simulink model "item2ModeloNLinPS"  (R2017a)
settings: Solver=VariableStepAuto  StartTime=0.0  StopTime=50  RelTol=1e-3
libraries: simulink x4
settings Model: Creator=julia  LastModifiedBy=julia

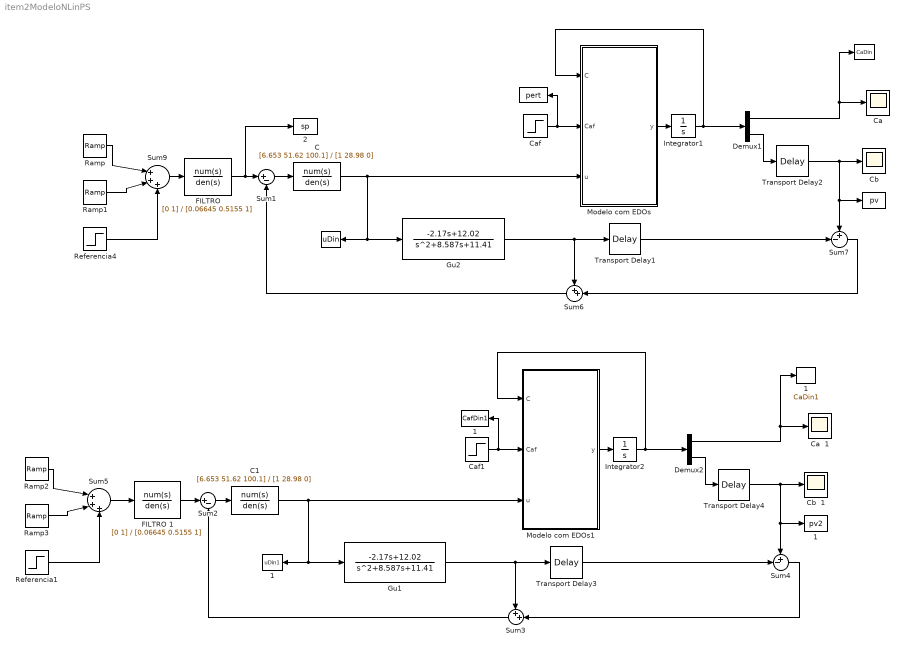
== system item2ModeloNLinPS ==
  "   " : ToWorkspace  VariableName=pv  SaveFormat=Timeseries  SampleTime=-1
  "          " : ToWorkspace  VariableName=pert  SaveFormat=Timeseries  SampleTime=-1
  "                 " : ToWorkspace  VariableName=uDin  SaveFormat=Timeseries  SampleTime=-1
  "                   " : ToWorkspace  VariableName=CaDin  SaveFormat=Timeseries  SampleTime=-1
  "                   1" : ToWorkspace  VariableName=CaDin1  SaveFormat=Timeseries  SampleTime=-1
  "                 1" : ToWorkspace  VariableName=uDin1  SaveFormat=Timeseries  SampleTime=-1
  "          1" : ToWorkspace  VariableName=CafDin1  SaveFormat=Timeseries  SampleTime=-1
  "   1" : ToWorkspace  VariableName=pv2  SaveFormat=Timeseries  SampleTime=-1
  "   2" : ToWorkspace  VariableName=sp  SaveFormat=Timeseries  SampleTime=-1
  C : TransferFcn  Numerator=[6.653 51.62 100.1]  Denominator=[1 28.98 0]
  C1 : TransferFcn  Numerator=[6.653 51.62 100.1]  Denominator=[1 28.98 0]
  "Ca  " : Scope
  Ca  1 : Scope
  Caf : Step  Time=40  Before=5.1  After=5.15  SampleTime=0
  Caf1 : Step  Time=40  Before=5.1  After=5.15  SampleTime=0
  "Cb  " : Scope
  Cb  1 : Scope
  Demux1 : Demux  Outputs=2
  Demux2 : Demux  Outputs=2
  "FILTRO " : TransferFcn  Numerator=[0 1]  Denominator=[0.06645 0.5155 1]
  FILTRO 1 : TransferFcn  Numerator=[0 1]  Denominator=[0.06645 0.5155 1]
  Gu1 : TransferFcn  Numerator=[-2.17 12.02]  Denominator=[1 8.587 11.41]
  Gu2 : TransferFcn  Numerator=[-2.17 12.02]  Denominator=[1 8.587 11.41]
  Integrator1 : Integrator  InitialCondition=[0;0]
  Integrator2 : Integrator  InitialCondition=[0;0]
  Modelo com EDOs : MATLAB Function  TreatAsAtomicUnit=on
  Modelo com EDOs1 : MATLAB Function  TreatAsAtomicUnit=on
  Ramp : simulink/Sources/Ramp  slope=2.345/10  start=0  X0=0
  Ramp1 : simulink/Sources/Ramp  slope=-2.345/10  start=10  X0=0
  Ramp2 : simulink/Sources/Ramp  slope=2.345/10  start=0  X0=0
  Ramp3 : simulink/Sources/Ramp  slope=-2.345/10  start=10  X0=0
  Referencia1 : Step  Time=30  After=0.35  SampleTime=0
  Referencia4 : Step  Time=30  After=0.1  SampleTime=0
  Sum1 : Sum  Inputs=|+-
  Sum2 : Sum  Inputs=|+-
  Sum3 : Sum  Inputs=++|
  Sum4 : Sum  Inputs=+-|
  Sum5 : Sum  Inputs=|+++
  Sum6 : Sum  Inputs=++|
  Sum7 : Sum  Inputs=+-|
  Sum9 : Sum  Inputs=|+++
  Transport Delay{1..4} (4 alike) : TransportDelay  DelayTime=3
  wires:
  Modelo com EDOs/1(y) -> Integrator1/1
  Integrator1/1 -> Modelo com EDOs/1(C), Demux1/1
  Demux1/1 -> "                   "/1, "Ca  "/1
  "FILTRO "/1 -> "   2"/1, Sum1/1
  Sum1/1 -> C/1
  Caf/1 -> "          "/1, Modelo com EDOs/2(Caf)
  Referencia4/1 -> Sum9/3
  Sum9/1 -> "FILTRO "/1
  Ramp1/1 -> Sum9/2
  Ramp/1 -> Sum9/1
  Gu2/1 -> Sum6/1, Transport Delay1/1
  Transport Delay1/1 -> Sum7/2
  Sum7/1 -> Sum6/2
  C/1 -> Modelo com EDOs/3(u), Gu2/1, "                 "/1
  Sum6/1 -> Sum1/2
  Demux1/2 -> Transport Delay2/1
  Transport Delay2/1 -> "   "/1, Sum7/1, "Cb  "/1
  Transport Delay4/1 -> Cb  1/1, Sum4/1, "   1"/1
  Demux2/2 -> Transport Delay4/1
  Sum3/1 -> Sum2/2
  C1/1 -> "                 1"/1, Gu1/1, Modelo com EDOs1/3(u)
  Sum4/1 -> Sum3/2
  Transport Delay3/1 -> Sum4/2
  Gu1/1 -> Transport Delay3/1, Sum3/1
  Ramp2/1 -> Sum5/1
  Ramp3/1 -> Sum5/2
  Sum5/1 -> FILTRO 1/1
  Referencia1/1 -> Sum5/3
  Caf1/1 -> Modelo com EDOs1/2(Caf), "          1"/1
  Sum2/1 -> C1/1
  FILTRO 1/1 -> Sum2/1
  Demux2/1 -> Ca  1/1, "                   1"/1
  Integrator2/1 -> Demux2/1, Modelo com EDOs1/1(C)
  Modelo com EDOs1/1(y) -> Integrator2/1

== matlab function item2ModeloNLinPS/Modelo com EDOs ==
  data: y output; C input; Caf input; u input
%EDOs das concentracoes dos produtos A e B
function y = fcn(C, Caf, u)

%constantes
k1 = 6.01; %L/min
k2 = 0.8433; %L/min
k3 = 0.1123; %mol/Lmin

%variaveis das concentracoes dos produtos A e B
Ca = C(1);
Cb = C(2);

%EDOs
Ca_d = -k1*Ca - k3*(Ca^2) + (Caf - Ca)*u;
Cb_d =  k1*Ca - k2*Cb - Cb*u;
 
%conjunto das EDOs
y = [Ca_d;Cb_d];

== matlab function item2ModeloNLinPS/Modelo com EDOs1 ==
  data: y output; C input; Caf input; u input
%EDOs das concentracoes dos produtos A e B
function y = fcn(C, Caf, u)

%constantes
k1 = 6.01; %L/min
k2 = 0.8433; %L/min
k3 = 0.1123; %mol/Lmin

%variaveis das concentracoes dos produtos A e B
Ca = C(1);
Cb = C(2);

%EDOs
Ca_d = -k1*Ca - k3*(Ca^2) + (Caf - Ca)*u;
Cb_d =  k1*Ca - k2*Cb - Cb*u;
 
%conjunto das EDOs
y = [Ca_d;Cb_d];
